simulink model "Modelo1"  (R2026a)
settings: Solver=VariableStepAuto
PreLoadFcn:
  | m = 1;
  | b = 2;
  | k = 1;
  | x0 = 0.1;
  | dx0 = 0;
settings Model: Creator=Alejandro  LastModifiedBy=Alejandro

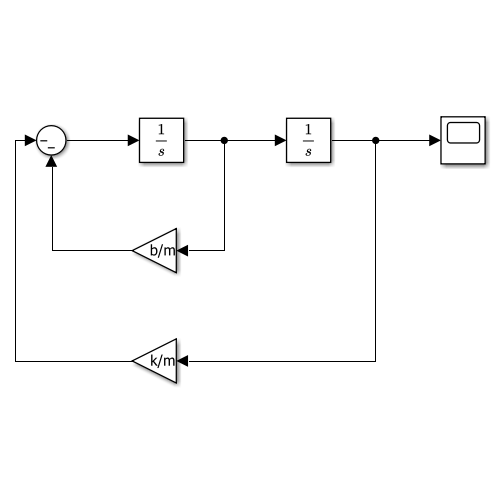
[thumbnail: Simulink's stored preview of the top-level diagram]
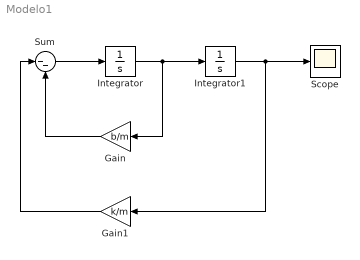
== system Modelo1 ==
  Gain : Gain  Gain=b/m
  Gain1 : Gain  Gain=k/m
  Integrator : Integrator  InitialCondition=dx0
  Integrator1 : Integrator  InitialCondition=x0
  Scope : Scope
      settings: ActiveDisplayYMinimum=-0.012443817557879775  ActiveDisplayYMaximum=0.11249375750643109
  Sum : Sum  Inputs=|--
  wires:
  Integrator/1 -> Gain/1, Integrator1/1
  Sum/1 -> Integrator/1
  Integrator1/1 -> Gain1/1, Scope/1
  Gain/1 -> Sum/2
  Gain1/1 -> Sum/1
